simulink library "CampusEnergyModeling"  (Simulink 8.1)
settings: Solver=ode45  StartTime=0.0  StopTime=10.0  RelTol=1e-3
undefined symbols (not defined in the file): a, b, c, j, look_Pin, look_Pout, magnitude
libraries: powerlib x6, simulink x3
(part 2 of 2)

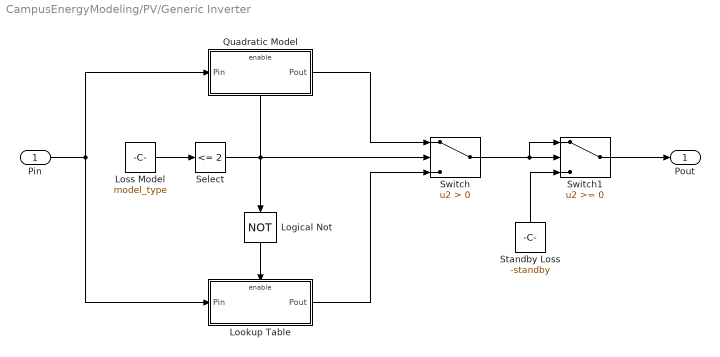
== system CampusEnergyModeling/PV/Generic Inverter ==
  Pin : Inport
  Logical Not : Logic  Operator=NOT  IconShape=distinctive  AllPortsSameDT=off  OutDataTypeStr=boolean
  Lookup Table : Subsystem  TreatAsAtomicUnit=on
  Loss Model : Constant  Value=model_type
  Quadratic Model : Subsystem  TreatAsAtomicUnit=on
  Select : simulink/Logic and Bit Operations/Compare To Constant  relop=<=  const=2  OutDataTypeStr=boolean
  Standby Loss : Constant  Value=-standby
  Switch : Switch  Criteria=u2 > Threshold  ZeroCross=off
  Switch1 : Switch  ZeroCross=off
  Pout : Outport
  wires:
  Loss Model/1 -> Select/1
  Logical Not/1 -> Lookup Table/Enable
  Pin/1 -> Quadratic Model/1(Pin), Lookup Table/1(Pin)
  Quadratic Model/1(Pout) -> Switch/1
  Select/1 -> Logical Not/1, Switch/2, Quadratic Model/Enable
  Lookup Table/1(Pout) -> Switch/3
  Switch/1 -> Switch1/1, Switch1/2
  Switch1/1 -> Pout/1
  Standby Loss/1 -> Switch1/3

== system CampusEnergyModeling/Weather/Weather Data ==
  From File : FromFile  FileName=TMY3.mat  OutDataTypeStr=Bus: BusDef_Weather  SampleTime=0  ExtrapolationBeforeFirstDataPoint=Hold first value  ExtrapolationAfterLastDataPoint=Hold last value
  Output : Outport  OutDataTypeStr=Bus: BusDef_Weather
  wires:
  From File/1 -> Output/1

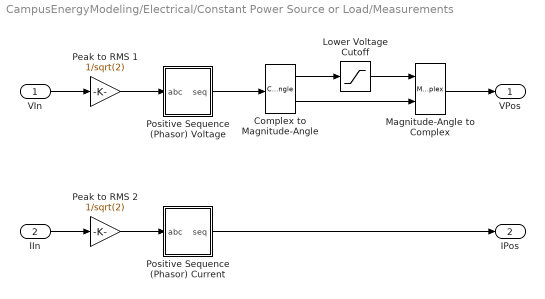
== system CampusEnergyModeling/Electrical/Constant Power Source or Load/Measurements ==
  VIn : Inport
  IIn : Inport  Port=2
  Complex to Magnitude-Angle : ComplexToMagnitudeAngle
  Lower Voltage Cutoff : Saturate  UpperLimit=inf  LowerLimit=VLow*VNom/sqrt(3)
  Magnitude-Angle to Complex : MagnitudeAngleToComplex
  Peak to RMS 1 : Gain  Gain=1/sqrt(2)
  Peak to RMS 2 : Gain  Gain=1/sqrt(2)
  Positive Sequence (Phasor) Current : Subsystem
      mask init:
      | j=sqrt(-1);
      | a=exp(j*2*pi/3);
      | a2=exp(-j*2*pi/3);
  Positive Sequence (Phasor) Voltage : Subsystem
      mask init:
      | j=sqrt(-1);
      | a=exp(j*2*pi/3);
      | a2=exp(-j*2*pi/3);
  VPos : Outport
  IPos : Outport  Port=2
  wires:
  Complex to Magnitude-Angle/2 -> Magnitude-Angle to Complex/2
  Lower Voltage Cutoff/1 -> Magnitude-Angle to Complex/1
  Magnitude-Angle to Complex/1 -> VPos/1
  Complex to Magnitude-Angle/1 -> Lower Voltage Cutoff/1
  Positive Sequence (Phasor) Voltage/1(seq) -> Complex to Magnitude-Angle/1
  Positive Sequence (Phasor) Current/1(seq) -> IPos/1
  Peak to RMS 2/1 -> Positive Sequence (Phasor) Current/1(abc)
  Peak to RMS 1/1 -> Positive Sequence (Phasor) Voltage/1(abc)
  IIn/1 -> Peak to RMS 2/1
  VIn/1 -> Peak to RMS 1/1

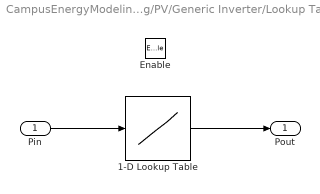
== system CampusEnergyModeling/PV/Generic Inverter/Lookup Table ==
  Pin : Inport
  Enable : EnablePort
  1-D Lookup Table : Lookup_n-D  NumberOfTableDimensions=1  BreakpointsForDimension1=look_Pin  IndexSearchMethod=Linear search  BeginIndexSearchUsingPreviousIndexResult=on  UseOneInputPortForAllInputData=on  Table=look_Pout  RndMeth=Simplest  InputSameDT=on
  Pout : Outport
  wires:
  Pin/1 -> 1-D Lookup Table/1
  1-D Lookup Table/1 -> Pout/1

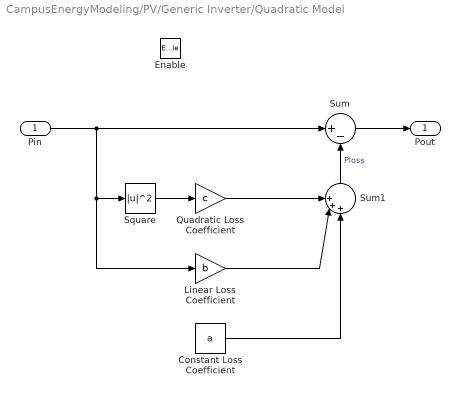
== system CampusEnergyModeling/PV/Generic Inverter/Quadratic Model ==
  Pin : Inport
  Enable : EnablePort
  Constant Loss Coefficient : Constant  Value=a
  Linear Loss Coefficient : Gain  Gain=b
  Quadratic Loss Coefficient : Gain  Gain=c
  Square : Math  Operator=magnitude^2  SaturateOnIntegerOverflow=on
  Sum : Sum  Inputs=|+-
  Sum1 : Sum  Inputs=+++||
  Pout : Outport
  wires:
  Pin/1 -> Sum/1, Linear Loss Coefficient/1, Square/1
  Square/1 -> Quadratic Loss Coefficient/1
  Quadratic Loss Coefficient/1 -> Sum1/1
  Sum/1 -> Pout/1
  Sum1/1 -> Sum/2  "Ploss"
  Linear Loss Coefficient/1 -> Sum1/2
  Constant Loss Coefficient/1 -> Sum1/3

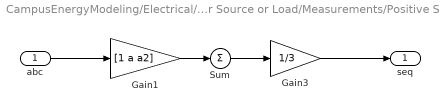
== system CampusEnergyModeling/Electrical/Constant Power Source or Load/Measurements/Positive Sequence (Phasor) Current ==
  abc : Inport
  Gain1 : Gain  Gain=[1 a a2]  SaturateOnIntegerOverflow=on  OutDataTypeStr=Inherit: Same as input  ParamDataTypeStr=Inherit: Same as input
  Gain3 : Gain  Gain=1/3  SaturateOnIntegerOverflow=on  OutDataTypeStr=Inherit: Same as input  ParamDataTypeStr=Inherit: Same as input
  Sum : Sum  Inputs=1  SaturateOnIntegerOverflow=on  InputSameDT=on  OutDataTypeStr=Inherit: Same as first input
  seq : Outport
  wires:
  Sum/1 -> Gain3/1
  Gain1/1 -> Sum/1
  Gain3/1 -> seq/1
  abc/1 -> Gain1/1

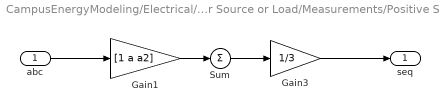
== system CampusEnergyModeling/Electrical/Constant Power Source or Load/Measurements/Positive Sequence (Phasor) Voltage ==
  abc : Inport
  Gain1 : Gain  Gain=[1 a a2]  SaturateOnIntegerOverflow=on  OutDataTypeStr=Inherit: Same as input  ParamDataTypeStr=Inherit: Same as input
  Gain3 : Gain  Gain=1/3  SaturateOnIntegerOverflow=on  OutDataTypeStr=Inherit: Same as input  ParamDataTypeStr=Inherit: Same as input
  Sum : Sum  Inputs=1  SaturateOnIntegerOverflow=on  InputSameDT=on  OutDataTypeStr=Inherit: Same as first input
  seq : Outport
  wires:
  Sum/1 -> Gain3/1
  Gain1/1 -> Sum/1
  Gain3/1 -> seq/1
  abc/1 -> Gain1/1
